simulink model "ssc_airvtol_elec_battery"  (R2026a)
settings: Solver=daessc  StopTime=2000  AbsTol=1e-3  EnableMultiTasking=on
PreLoadFcn:
  | ssc_airvtol_elec_default_params
  | battery_capacity = 180;battery_pdensity = 240;payload_mass_workspace = 80;
PostLoadFcn:
  | warning('off','physmod:common:gl:sli:rtp:InvalidNonValueReference');
  | warning off Simulink:Engine:SortDiscontinuityInAlgLoop
model workspace (MATLAB code in the model file):
  | v0                 = 0; % Initial vehicle speed
  | wheel_radius = 0.15; % Wheel radius
  | k                   = 1e-2; % Motor losses (W/(N*M)^2)
  | t_torque        = 0.02; % Electric motor time constant
  | rpm0             = 2000; % Engine initial speed demand
undefined symbols (not defined in the file): battery_vnom, propeller_num
libraries: fl_lib x49, nesl_utility x13, ee_lib x12, ssc_airvtol_components x11, sdl_lib x8, simulink x6, batteryecm_lib x2, pack_5p48s8p_Thr_library x2, pack_5p48s8p_1g10g1_5g1g5_Thr_library x1, pack_5p48s8p_1g10g1_Iso_library x1, pack_5p48s8p_1g10g1_Thr_library x1, pack_5p48s8p_4g4g4_Iso_library x1
(part 2 of 2)

== system ssc_airvtol_elec_battery/Battery/Abstract ==
  Battery : batteryecm_lib/Battery  Vnom=201.6 V  prm_dir=1  R1_dis=2 Ohm  R1_ch=2 Ohm  R1=0.05 Ohm  prm_AH=2  AH=battery_capacity hr*A  V1=163 V  AH1=0.25*battery_capacity hr*A  prm_R2=1  R2=2000 Ohm  Tmeas=298.15 K  charge_measurement_port=simscape.enum.battery.enable.yes  prm_dyn=1  Rp1=0.005 Ohm  tau1=30 s  Rp2=0.005 Ohm  tau2=30 s  Rp3=0.005 Ohm  tau3=30 s  Rp4=0.005 Ohm  tau4=30 s  Rp5=0.005 Ohm  tau5=30 s  prm_fade=1  N_fade=100  AH_fade=45 hr*A  R1_fade=2.02 Ohm  R1_ch_fade=2.02 Ohm  V1_fade=10.35 V  prm_age=1  prm_age_OCV=1  OCV_age=0.9  SOC_age=60  Tmeas_age=298.15 K  delta_time_age_vec=[0] d  temperature_age_vec=[273] K  OCV_scaling_age=2.2134e6  OCV_offset_age=1.632e6  temp_exp_age=0.515833569 V  t_exp_age=0.75  Vnom_T2=12 V  R1_T2=2.2 Ohm  R1_T2_dis=2.2 Ohm  R1_T2_ch=2.2 Ohm  V1_T2=11.4 V  R2_T2=2200 Ohm  Rp1_T2=0.005 Ohm  tau1_T2=30 s  Rp2_T2=0.005 Ohm  tau2_T2=30 s  Rp3_T2=0.005 Ohm  tau3_T2=30 s  Rp4_T2=0.005 Ohm  tau4_T2=30 s  Rp5_T2=0.005 Ohm  tau5_T2=30 s  Tmeas2=273.15 K  thermal_port=simscape.enum.thermaleffects.omit  thermal_mass=30000 J/K  i_specify=off  i_priority=None  i=0 A  i_nominal_specify=off  i_nominal_value=1  i_nominal_unit=A  v_specify=off  v_priority=None  v=0 V  v_nominal_specify=off  v_nominal_value=1  v_nominal_unit=V  charge_specify=on  charge_priority=High  charge=battery_capacity hr*A  charge_nominal_specify=off  charge_nominal_value=1  charge_nominal_unit=A*hr  num_cycles_specify=off  num_cycles_priority=High  num_cycles=0  num_cycles_nominal_specify=off  num_cycles_nominal_value=1  num_cycles_nominal_unit=1  temperature_specify=off  temperature_priority=High  temperature=298.15 K  temperature_nominal_specify=off  temperature_nominal_value=1  temperature_nominal_unit=K
  Gain : Gain  Gain=1/battery_capacity
  PS-Simulink Converter : nesl_utility/PS-Simulink Converter  PhysicalDomain=network_engine_domain  SubClassName=ps_output  LeftPortType=input  RightPortType=output  PseudoPeriodic=off  Frequencies=[]  VectorFormat=1-D array  Unit=A*hr  AffineConversion=off
  + : PMIOPort  Side=Right
  - : PMIOPort  Port=2  Side=Left
  SOC : Outport
  wires:
  PS-Simulink Converter/1 -> Gain/1
  Gain/1 -> SOC/1
  connections:
  Battery/RConn1 -- -/RConn1
  Battery/LConn1 -- +/RConn1
  Battery/LConn2 -- PS-Simulink Converter/LConn1

== system ssc_airvtol_elec_battery/Battery/DetEdge Plate ==
  Ambient Temperature : fl_lib/Thermal/Thermal Sources/Temperature Source  temperature=298 K
  Bus Selector : BusSelector  OutputSignals=A1.socC.M1
  Constant : Constant
  Pack : pack_5p48s8p_1g10g1_5g1g5_Thr_library/Pack  cell_param=ModuleType1  targets=targets_5p48s8p_1g10g1_5g1g5_thr  plate=plate_5p48s_1g10g1_5g1g5_thr  batt_obj=batt_5p48s_1g10g1_5g1g5_thr
  + : PMIOPort  Side=Right
  - : PMIOPort  Port=2  Side=Left
  SOC : Outport
  wires:
  Bus Selector/1 -> SOC/1  "<M1>"
  Pack/1 -> Bus Selector/1
  Constant/1 -> Pack/1
  connections:
  +/RConn1 -- Pack/LConn1
  -/RConn1 -- Pack/RConn1
  Ambient Temperature/LConn1 -- Pack/RConn2

== system ssc_airvtol_elec_battery/Battery/Edges Iso ==
  Bus Selector : BusSelector  OutputSignals=A1.socC.M1
  Constant : Constant
  Min : MinMax
  Pack : pack_5p48s8p_1g10g1_Iso_library/Pack  cell_param=ModuleType1  targets=targets_5p48s8p_1g10g1_iso  plate=plate_5p48s_1g10g1_thr  batt_obj=batt_5p48s_1g10g1_thr
  + : PMIOPort  Side=Right
  - : PMIOPort  Port=2  Side=Left
  SOC : Outport
  wires:
  Min/1 -> SOC/1
  Pack/1 -> Bus Selector/1
  Constant/1 -> Pack/1
  Bus Selector/1 -> Min/1  "<M1>"
  connections:
  -/RConn1 -- Pack/RConn1
  +/RConn1 -- Pack/LConn1

== system ssc_airvtol_elec_battery/Battery/Edges Plate ==
  Ambient Temperature : fl_lib/Thermal/Thermal Sources/Temperature Source  temperature=298 K
  Bus Selector : BusSelector  OutputSignals=A1.socC.M1
  Constant : Constant
  Pack : pack_5p48s8p_1g10g1_Thr_library/Pack  cell_param=ModuleType1  targets=targets_5p48s8p_1g10g1_thr  plate=plate_5p48s_1g10g1_thr  batt_obj=batt_5p48s_1g10g1_thr
  + : PMIOPort  Side=Right
  - : PMIOPort  Port=2  Side=Left
  SOC : Outport
  wires:
  Bus Selector/1 -> SOC/1  "<M1>"
  Pack/1 -> Bus Selector/1
  Constant/1 -> Pack/1
  connections:
  Pack/LConn1 -- +/RConn1
  Pack/RConn1 -- -/RConn1
  Ambient Temperature/LConn1 -- Pack/RConn2

== system ssc_airvtol_elec_battery/Battery/Equal Iso ==
  Bus Selector : BusSelector  OutputSignals=A1.socC.M1
  Constant : Constant
  Min : MinMax
  Pack : pack_5p48s8p_4g4g4_Iso_library/Pack  cell_param=ModuleType1  targets=targets_5p48s8p_4g4g4_iso
  + : PMIOPort  Side=Right
  - : PMIOPort  Port=2  Side=Left
  SOC : Outport
  wires:
  Min/1 -> SOC/1
  Pack/1 -> Bus Selector/1
  Constant/1 -> Pack/1
  Bus Selector/1 -> Min/1  "<M1>"
  connections:
  +/RConn1 -- Pack/LConn1
  -/RConn1 -- Pack/RConn1

== system ssc_airvtol_elec_battery/Battery/Equal Plate ==
  Ambient Temperature : fl_lib/Thermal/Thermal Sources/Temperature Source  temperature=298 K
  Bus Selector : BusSelector  OutputSignals=A1.socC.M1
  Constant : Constant
  Pack : pack_5p48s8p_4g4g4_Thr_library/Pack  cell_param=ModuleType1  targets=targets_5p48s8p_4g4g4_thr  plate=plate_5p48s_4g4g4_thr  batt_obj=batt_5p48s_4g4g4_thr
  + : PMIOPort  Side=Right
  - : PMIOPort  Port=2  Side=Left
  SOC : Outport
  wires:
  Constant/1 -> Pack/1
  Bus Selector/1 -> SOC/1  "<M1>"
  Pack/1 -> Bus Selector/1
  connections:
  -/RConn1 -- Pack/RConn1
  +/RConn1 -- Pack/LConn1
  Ambient Temperature/LConn1 -- Pack/RConn2

== system ssc_airvtol_elec_battery/Battery/Lumped BCs ==
  Ambient Temperature : fl_lib/Thermal/Thermal Sources/Temperature Source  temperature=298 K
  Bus Selector : BusSelector  OutputSignals=A1.socC.M1
  Constant : Constant
  Pack : pack_5p48s8p_Thr_library/Pack Simple Cooling  cell_param=ModuleType1  targets=targets_5p48s8p_thr  batt_obj=batt_5p48s_thr  coolant_temp=[23 26]
  + : PMIOPort  Side=Right
  - : PMIOPort  Port=2  Side=Left
  SOC : Outport
  wires:
  Constant/1 -> Pack/1
  Bus Selector/1 -> SOC/1  "<M1>"
  Pack/1 -> Bus Selector/1
  connections:
  Pack/LConn1 -- +/RConn1
  Pack/RConn1 -- -/RConn1
  Pack/RConn2 -- Ambient Temperature/LConn1

== system ssc_airvtol_elec_battery/Battery/Lumped Plate ==
  Ambient Temperature : fl_lib/Thermal/Thermal Sources/Temperature Source  temperature=298 K
  Bus Selector : BusSelector  OutputSignals=A1.socC.M1
  Constant : Constant
  Pack : pack_5p48s8p_Thr_library/Pack  cell_param=ModuleType1  targets=targets_5p48s8p_thr  plate=plate_5p48s_thr  batt_obj=batt_5p48s_thr
  + : PMIOPort  Side=Right
  - : PMIOPort  Port=2  Side=Left
  SOC : Outport
  wires:
  Pack/1 -> Bus Selector/1
  Bus Selector/1 -> SOC/1  "<M1>"
  Constant/1 -> Pack/1
  connections:
  Pack/RConn2 -- Ambient Temperature/LConn1
  Pack/RConn1 -- -/RConn1
  +/RConn1 -- Pack/LConn1

== system ssc_airvtol_elec_battery/Battery/Specific ==
  Add cells in series VCVS : fl_lib/Electrical/Electrical Sources/Voltage-Controlled Voltage Source  K=4*12-1  v1_specify=off  v1_priority=None  v1=0 V  v1_nominal_specify=off  v1_nominal_value=1  v1_nominal_unit=V  v2_specify=off  v2_priority=None  v2=0 V  v2_nominal_specify=off  v2_nominal_value=1  v2_nominal_unit=V
  Add strings in parallel CCCS : fl_lib/Electrical/Electrical Sources/Current-Controlled Current Source  K=5*8-1  i1_specify=off  i1_priority=None  i1=0 A  i1_nominal_specify=off  i1_nominal_value=1  i1_nominal_unit=A  i2_specify=off  i2_priority=None  i2=0 A  i2_nominal_specify=off  i2_nominal_value=1  i2_nominal_unit=A
  Ambient Temperature : fl_lib/Thermal/Thermal Sources/Temperature Source  temperature=298 K
  Battery (Table-Based) : batteryecm_lib/Battery (Table-Based)  SOC_vec=batteryTableBased.parameters.SOC_vec.value  T_dependence=simscape.enum.tablebattery.temperature_dependence.yes  prm_dir=simscape.enum.tablebattery.prm_dir.noCurrentDirectionality  T_vec=batteryTableBased.parameters.T_vec.value degC  V0_mat=batteryTableBased.parameters.V0_mat.value V  V0_vec=batteryTableBased.parameters.V0_vec.value V  V_range=[0, inf] V  R0_mat=batteryTableBased.parameters.R0_mat.value Ohm  R0_vec=batteryTableBased.parameters.R0_vec.value Ohm  R0_dis_mat=[.0117, .0085, .009; .011, .0085, .009; .0114, .0087, .0092; .0107, .0082, .0088; .0107, .0083, .0091; .0113, .0085, .0089; .0116, .0085, .0089] Ohm  R0_dis_vec=[.0085, .0085, .0087, .0082, .0083, .0085, .0085] Ohm  R0_ch_mat=[.0117, .0085, .009; .011, .0085, .009; .0114, .0087, .0092; .0107, .0082, .0088; .0107, .0083, .0091; .0113, .0085, .0089; .0116, .0085, .0089] Ohm  R0_ch_vec=[.0085, .0085, .0087, .0082, .0083, .0085, .0085] Ohm  AH=batteryTableBased.parameters.AH.value A*hr  prm_leak=simscape.enum.tablebattery.prm_leak.disabled  Rleak_vec=[8000, 7000, 6000] Ohm  Rleak=7e3 Ohm  extrapolation_option=simscape.enum.extrapolation.nearest  SOC_port=simscape.enum.tablebattery.enable.yes  prm_dyn=simscape.enum.tablebattery.prm_dyn.off  R1_mat=[.0109, .0029, .0013; .0069, .0024, .0012; .0047, .0026, .0013; .0034, .0016, .001; .0033, .0023, .0014; .0033, .0018, .0011; .0028, .0017, .0011] Ohm  R1_vec=[.0029, .0024, .0026, .0016, .0023, .0018, .0017] Ohm  tau1_mat=[20, 36, 39; 31, 45, 39; 109, 105, 61; 36, 29, 26; 59, 77, 67; 40, 33, 29; 25, 39, 33] s  tau1_vec=[36, 45, 105, 29, 77, 33, 39] s  R2_mat=[.0109, .0029, .0013; .0069, .0024, .0012; .0047, .0026, .0013; .0034, .0016, .001; .0033, .0023, .0014; .0033, .0018, .0011; .0028, .0017, .0011] Ohm  R2_vec=[.0029, .0024, .0026, .0016, .0023, .0018, .0017] Ohm  tau2_mat=[20, 36, 39; 31, 45, 39; 109, 105, 61; 36, 29, 26; 59, 77, 67; 40, 33, 29; 25, 39, 33] s  tau2_vec=[36, 45, 105, 29, 77, 33, 39] s  R3_mat=[.0109, .0029, .0013; .0069, .0024, .0012; .0047, .0026, .0013; .0034, .0016, .001; .0033, .0023, .0014; .0033, .0018, .0011; .0028, .0017, .0011] Ohm  R3_vec=[.0029, .0024, .0026, .0016, .0023, .0018, .0017] Ohm  tau3_mat=[20, 36, 39; 31, 45, 39; 109, 105, 61; 36, 29, 26; 59, 77, 67; 40, 33, 29; 25, 39, 33] s  tau3_vec=[36, 45, 105, 29, 77, 33, 39] s  R4_mat=[.0109, .0029, .0013; .0069, .0024, .0012; .0047, .0026, .0013; .0034, .0016, .001; .0033, .0023, .0014; .0033, .0018, .0011; .0028, .0017, .0011] Ohm  R4_vec=[.0029, .0024, .0026, .0016, .0023, .0018, .0017] Ohm  tau4_mat=[20, 36, 39; 31, 45, 39; 109, 105, 61; 36, 29, 26; 59, 77, 67; 40, 33, 29; 25, 39, 33] s  tau4_vec=[36, 45, 105, 29, 77, 33, 39] s  R5_mat=[.0109, .0029, .0013; .0069, .0024, .0012; .0047, .0026, .0013; .0034, .0016, .001; .0033, .0023, .0014; .0033, .0018, .0011; .0028, .0017, .0011] Ohm  R5_vec=[.0029, .0024, .0026, .0016, .0023, .0018, .0017] Ohm  tau5_mat=[20, 36, 39; 31, 45, 39; 109, 105, 61; 36, 29, 26; 59, 77, 67; 40, 33, 29; 25, 39, 33] s  tau5_vec=[36, 45, 105, 29, 77, 33, 39] s  prm_fade=simscape.enum.tablebattery.prm_fade.disabled  N0=100  dV0=0  dR0=0  dAH=0  dRleak=0  dR1=0  dR2=0  dR3=0  dR4=0  dR5=0  N0vec=[100, 200, 300]  Tfadevec=[298.15, 323.15] K  dV0vec=[0, 0, 0]  dR0vec=[0, 0, 0]  dAHvec=[0, 0, 0]  dRleakvec=[0, 0, 0]  dR1vec=[0, 0, 0]  dR2vec=[0, 0, 0]  dR3vec=[0, 0, 0]  dR4vec=[0, 0, 0]  dR5vec=[0, 0, 0]  dV0mat=[0, 0; 0, 0; 0, 0]  dR0mat=[0, 0; 0, 0; 0, 0]  dAHmat=[0, 0; 0, 0; 0, 0]  dRleakmat=[0, 0; 0, 0; 0, 0]  dR1mat=[0, 0; 0, 0; 0, 0]  dR2mat=[0, 0; 0, 0; 0, 0]  dR3mat=[0, 0; 0, 0; 0, 0]  dR4mat=[0, 0; 0, 0; 0, 0]  dR5mat=[0, 0; 0, 0; 0, 0]  prm_age_modeling=simscape.enum.tablebattery.prm_age_modeling.equation  storage_dt_age_vec=[0] d  storage_T_age_vec=[273] K  prm_age_OCV=simscape.enum.tablebattery.prm_age_OCV.OCV  OCV_age=0.9  SOC_age=0.6  prm_age_resistance=simscape.enum.tablebattery.prm_age.disabled  OCV_scaling_age_resistance=2.2134e6  OCV_offset_age_resistance=1.632e6  temp_exp_age_resistance=0.515833569 V  t_exp_age_resistance=0.75  T_age_vec_resistance=[273.15, 298.15, 323.15] K  dt_age_vec_resistance=[90, 180, 270, 360] d  dR0_age_vec=[0, 0, 0]  t_meas_dR0_age=100 d  dR0_age_mat=[0, 0, 0; 0, 0, 0; 0, 0, 0; 0, 0, 0]  prm_age_capacity=simscape.enum.tablebattery.prm_age.disabled  OCV_scaling_age_capacity=1.5097e07  OCV_offset_age_capacity=8.3625e06  temp_exp_age_capacity=0.6011 V  t_exp_age_capacity=0.75  T_age_vec_capacity=[273.15, 298.15, 323.15] K  dt_age_vec_capacity=[90, 180, 270, 360] d  dAH_age_vec=[0, 0, 0]  t_meas_dAH_age=100 d  dAH_age_mat=[0, 0, 0; 0, 0, 0; 0, 0, 0; 0, 0, 0]  thermal_port=simscape.enum.thermaleffects.model  temperature=298.15 K  thermal_mass=100 J/K  i_specify=off  i_priority=None  i=0 A  i_nominal_specify=off  i_nominal_value=1  i_nominal_unit=A  v_specify=off  v_priority=None  v=0 V  v_nominal_specify=off  v_nominal_value=1  v_nominal_unit=V  stateOfCharge_specify=on  stateOfCharge_priority=High  stateOfCharge=0.995  stateOfCharge_nominal_specify=off  stateOfCharge_nominal_value=1  stateOfCharge_nominal_unit=1  num_cycles_specify=off  num_cycles_priority=High  num_cycles=0  num_cycles_nominal_specify=off  num_cycles_nominal_value=1  num_cycles_nominal_unit=1  cell_temperature_specify=on  cell_temperature_priority=None  cell_temperature=298.15 K  cell_temperature_nominal_specify=off  cell_temperature_nominal_value=1  cell_temperature_nominal_unit=K
  PS-Simulink Converter : nesl_utility/PS-Simulink Converter  PhysicalDomain=network_engine_domain  SubClassName=ps_output  LeftPortType=input  RightPortType=output  PseudoPeriodic=off  Frequencies=[]  VectorFormat=1-D array  Unit=A*hr  AffineConversion=off
  + : PMIOPort  Side=Right
  - : PMIOPort  Port=2  Side=Left
  SOC : Outport
  wires:
  PS-Simulink Converter/1 -> SOC/1
  connections:
  Battery (Table-Based)/LConn2 -- PS-Simulink Converter/LConn1
  -/RConn1 -- Add cells in series VCVS/RConn1 -- Battery (Table-Based)/RConn1 -- Add strings in parallel CCCS/RConn2
  +/RConn1 -- Add strings in parallel CCCS/LConn2 -- Add strings in parallel CCCS/RConn1
  Add cells in series VCVS/LConn1 -- Battery (Table-Based)/LConn1 -- Add cells in series VCVS/RConn2
  Add strings in parallel CCCS/LConn1 -- Add cells in series VCVS/LConn2
  Ambient Temperature/LConn1 -- Battery (Table-Based)/RConn2

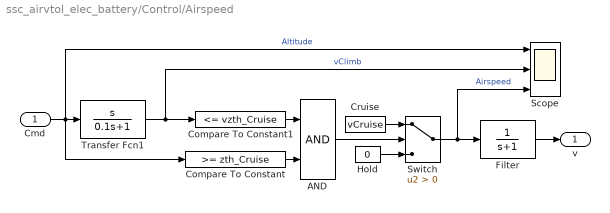
== system ssc_airvtol_elec_battery/Control/Airspeed ==
  Cmd : Inport
  AND : Logic  AllPortsSameDT=off  OutDataTypeStr=boolean
  Compare To Constant : simulink/Logic and Bit Operations/Compare To Constant  relop=>=  const=zth_Cruise  OutDataTypeStr=boolean
  Compare To Constant1 : simulink/Logic and Bit Operations/Compare To Constant  relop=<=  const=vzth_Cruise  OutDataTypeStr=boolean
  Cruise : Constant  Value=vCruise
  Filter : TransferFcn  Denominator=[1 1]
  Hold : Constant  Value=0
  Scope : Scope  NumInputPorts=3
      settings: ActiveDisplayYMinimum=-12.5  ActiveDisplayYMaximum=112.5  DataLoggingVariableName=ScopeData2
  Switch : Switch  Criteria=u2 > Threshold  SaturateOnIntegerOverflow=off  InputSameDT=off
  Transfer Fcn1 : TransferFcn  Numerator=[1 0]  Denominator=[0.1 1]
  v : Outport
  wires:
  Compare To Constant/1 -> AND/2
  Switch/1 -> Scope/3, Filter/1  "Airspeed"
  Compare To Constant1/1 -> AND/1
  AND/1 -> Switch/2
  Transfer Fcn1/1 -> Scope/2, Compare To Constant1/1  "vClimb"
  Cruise/1 -> Switch/1
  Cmd/1 -> Compare To Constant/1, Scope/1, Transfer Fcn1/1  "Altitude"
  Hold/1 -> Switch/3
  Filter/1 -> v/1

== system ssc_airvtol_elec_battery/DC Power Distribution/Mux ==
  Cmd : Inport
  Demux : Demux  Outputs=3
  Simulink-PS Converter1 : nesl_utility/Simulink-PS Converter  PhysicalDomain=network_engine_domain  SubClassName=ps_input  LeftPortType=input  RightPortType=output  PseudoPeriodic=off  Frequencies=[]  NoiseDistribution=none  NoiseParameters=[]  Unit=1  AffineConversion=off  FilteringAndDerivatives=zero  SimscapeFilterOrder=1  InputFilterTimeConstant=0.005  UdotUserProvided=1
  Simulink-PS Converter5 : nesl_utility/Simulink-PS Converter  PhysicalDomain=network_engine_domain  SubClassName=ps_input  LeftPortType=input  RightPortType=output  PseudoPeriodic=off  Frequencies=[]  NoiseDistribution=none  NoiseParameters=[]  Unit=1  AffineConversion=off  FilteringAndDerivatives=zero  SimscapeFilterOrder=1  InputFilterTimeConstant=0.005  UdotUserProvided=1
  Simulink-PS Converter6 : nesl_utility/Simulink-PS Converter  PhysicalDomain=network_engine_domain  SubClassName=ps_input  LeftPortType=input  RightPortType=output  PseudoPeriodic=off  Frequencies=[]  NoiseDistribution=none  NoiseParameters=[]  Unit=1  AffineConversion=off  FilteringAndDerivatives=zero  SimscapeFilterOrder=1  InputFilterTimeConstant=0.005  UdotUserProvided=1
  Lamp : PMIOPort  Side=Right
  Heat : PMIOPort  Port=2  Side=Right
  Avioincs : PMIOPort  Port=3  Side=Right
  wires:
  Demux/1 -> Simulink-PS Converter6/1
  Demux/2 -> Simulink-PS Converter5/1
  Demux/3 -> Simulink-PS Converter1/1
  Cmd/1 -> Demux/1
  connections:
  Simulink-PS Converter5/RConn1 -- Heat/RConn1
  Simulink-PS Converter6/RConn1 -- Lamp/RConn1
  Simulink-PS Converter1/RConn1 -- Avioincs/RConn1

== system ssc_airvtol_elec_battery/DC Power Distribution/Sensing Current ==
  Current Sensor : fl_lib/Electrical/Electrical Sensors/Current Sensor
  PS-Simulink Converter1 : nesl_utility/PS-Simulink Converter  PhysicalDomain=network_engine_domain  SubClassName=ps_output  LeftPortType=input  RightPortType=output  PseudoPeriodic=off  Frequencies=[]  VectorFormat=1-D array  Unit=1  AffineConversion=off
  + : PMIOPort  Side=Left
  - : PMIOPort  Port=2  Side=Right
  i : Outport
  wires:
  PS-Simulink Converter1/1 -> i/1
  connections:
  Current Sensor/RConn2 -- -/RConn1
  Current Sensor/LConn1 -- +/RConn1
  Current Sensor/RConn1 -- PS-Simulink Converter1/LConn1

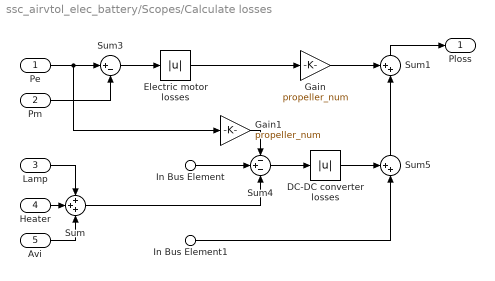
== system ssc_airvtol_elec_battery/Scopes/Calculate losses ==
  Pe : Inport
  Pm : Inport  Port=2
  Lamp : Inport  Port=3
  Heater : Inport  Port=4
  Avi : Inport  Port=5
  In Bus Element : Inport  Port=6  PortName=Batt  Element=Pe
  In Bus Element1 : Inport  Port=6  PortName=Batt  Element=Po
  " Electric motor losses" : Abs
  DC-DC converter losses : Abs
  Gain : Gain  Gain=propeller_num
  Gain1 : Gain  Gain=propeller_num
  Sum : Sum  Inputs=+++
  Sum1 : Sum  Inputs=++|
  Sum3 : Sum  Inputs=|+-
  Sum4 : Sum  Inputs=-+-
  Sum5 : Sum  Inputs=++|
  Ploss : Outport  VectorParamsAs1DForOutWhenUnconnected=off
  wires:
  In Bus Element1/1 -> Sum5/2
  DC-DC converter losses/1 -> Sum5/1
  " Electric motor losses"/1 -> Gain/1
  Pe/1 -> Gain1/1, Sum3/1
  In Bus Element/1 -> Sum4/2
  Sum5/1 -> Sum1/2
  Sum4/1 -> DC-DC converter losses/1
  Sum3/1 -> " Electric motor losses"/1
  Pm/1 -> Sum3/2
  Sum1/1 -> Ploss/1
  Lamp/1 -> Sum/1
  Heater/1 -> Sum/2
  Avi/1 -> Sum/3
  Gain/1 -> Sum1/1
  Gain1/1 -> Sum4/1
  Sum/1 -> Sum4/3

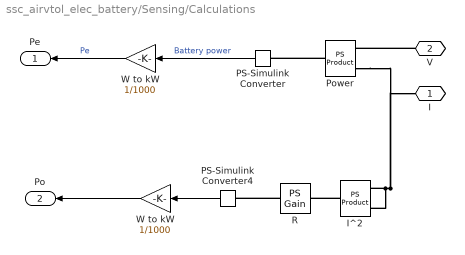
== system ssc_airvtol_elec_battery/Sensing/Calculations ==
  " W to kW " : Gain  Gain=1/1000
  I^2 : fl_lib/Physical Signals/Functions/PS Product
  PS-Simulink Converter : nesl_utility/PS-Simulink Converter  PhysicalDomain=network_engine_domain  SubClassName=ps_output  LeftPortType=input  RightPortType=output  PseudoPeriodic=off  Frequencies=[]  VectorFormat=1-D array  Unit=W  AffineConversion=off
  PS-Simulink Converter4 : nesl_utility/PS-Simulink Converter  PhysicalDomain=network_engine_domain  SubClassName=ps_output  LeftPortType=input  RightPortType=output  PseudoPeriodic=off  Frequencies=[]  VectorFormat=1-D array  Unit=W  AffineConversion=off
  Power : fl_lib/Physical Signals/Functions/PS Product
  R : fl_lib/Physical Signals/Functions/PS Gain  gain=0.05 Ohm
  W to kW : Gain  Gain=1/1000
  I : PMIOPort  Side=Left
  V : PMIOPort  Port=2  Side=Left
  Pe : Outport
  Po : Outport  Port=2
  wires:
  " W to kW "/1 -> Po/1
  PS-Simulink Converter4/1 -> " W to kW "/1
  W to kW/1 -> Pe/1  "Pe"
  PS-Simulink Converter/1 -> W to kW/1  "Battery power"
  connections:
  R/RConn1 -- PS-Simulink Converter4/LConn1
  I^2/RConn1 -- R/LConn1
  I^2/LConn1 -- I/RConn1 -- Power/LConn2 -- I^2/LConn2
  V/RConn1 -- Power/LConn1
  Power/RConn1 -- PS-Simulink Converter/LConn1

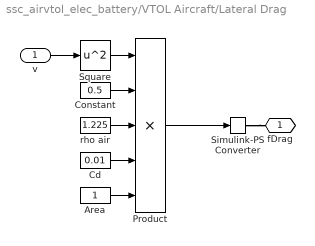
== system ssc_airvtol_elec_battery/VTOL Aircraft/Lateral Drag ==
  v : Inport
  Area : Constant
  Cd : Constant  Value=0.01
  Constant : Constant  Value=0.5
  Product : Product  Inputs=5
  Simulink-PS Converter : nesl_utility/Simulink-PS Converter  PhysicalDomain=network_engine_domain  SubClassName=ps_input  LeftPortType=input  RightPortType=output  PseudoPeriodic=off  Frequencies=[]  NoiseDistribution=none  NoiseParameters=[]  Unit=N  AffineConversion=off  FilteringAndDerivatives=filter  SimscapeFilterOrder=1  InputFilterTimeConstant=0.1  UdotUserProvided=0
  Square : Math  Operator=square
  rho air : Constant  Value=1.225
  fDrag : PMIOPort  Side=Right
  wires:
  v/1 -> Square/1
  Square/1 -> Product/1
  Constant/1 -> Product/2
  rho air/1 -> Product/3
  Cd/1 -> Product/4
  Product/1 -> Simulink-PS Converter/1
  Area/1 -> Product/5
  connections:
  Simulink-PS Converter/RConn1 -- fDrag/RConn1
